simulink model "Q15"  (R2016b)
settings: Solver=VariableStepAuto  StartTime=0.0  StopTime=10.0  RelTol=1e-3
libraries: simulink x1
settings Model: Creator=AKSHAY JP PAWAR  LastModifiedBy=AKSHAY JP PAWAR
settings DataIOCC: ReturnWorkspaceOutputs=on
settings SFSimCC: SimUseLocalCustomCode=on
settings RTWCC: RTWUseLocalCustomCode=on

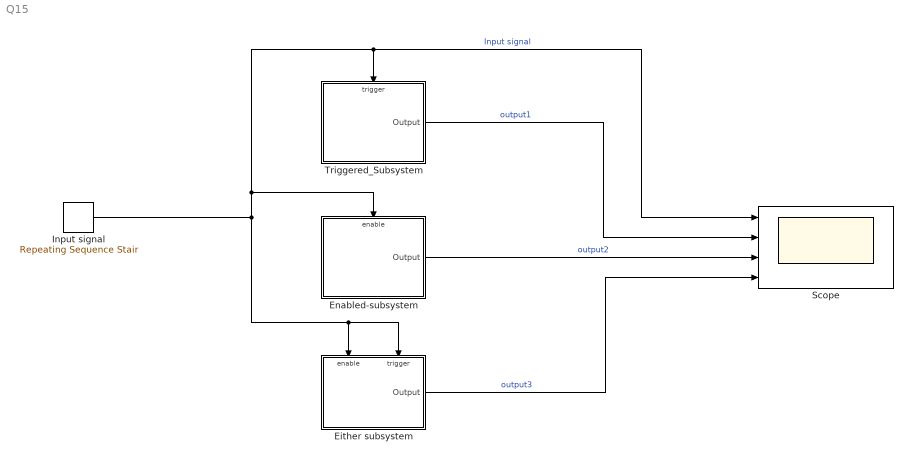
== system Q15 ==
  Either subsystem : Subsystem
  Enabled-subsystem : Subsystem
  Input signal : simulink/Sources/Repeating Sequence Stair  OutValues=[0 1 1 0 0].'  tsamp=-1  OutMin=[]  OutMax=[]  OutDataTypeStr=double  OutputDataTypeScalingMode=double  OutDataType=fixdt(0,8)  ConRadixGroup=Best Precision: Vector-wise  OutScaling=2^-12
  Scope : Scope  NumInputPorts=4
  Triggered_Subsystem : Subsystem
  wires:
  Triggered_Subsystem/1(Output) -> Scope/2  "output1"
  Enabled-subsystem/1(Output) -> Scope/3  "output2"
  Either subsystem/1(Output) -> Scope/4  "output3"
  Input signal/1 -> Enabled-subsystem/Enable, Triggered_Subsystem/Trigger, Scope/1, Either subsystem/Enable, Either subsystem/Trigger  "Input signal"

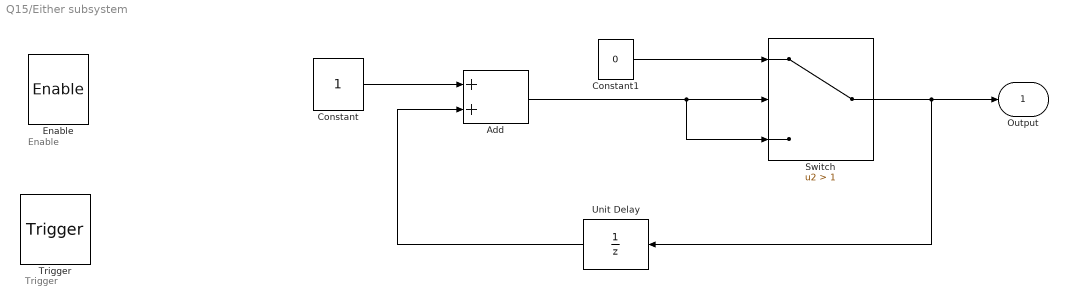
== system Q15/Either subsystem ==
  note: Trigger
  note: Enable
  Enable : EnablePort
  Trigger : TriggerPort  VariantControl=Variant  PortDimensions=1
  Add : Sum
  Constant : Constant
  Constant1 : Constant  Value=0
  Switch : Switch  Criteria=u2 > Threshold  Threshold=1
  Unit Delay : UnitDelay  SampleTime=-1  HasFrameUpgradeWarning=on
  Output : Outport
  wires:
  Add/1 -> Switch/3, Switch/2
  Unit Delay/1 -> Add/2
  Constant/1 -> Add/1
  Constant1/1 -> Switch/1
  Switch/1 -> Unit Delay/1, Output/1

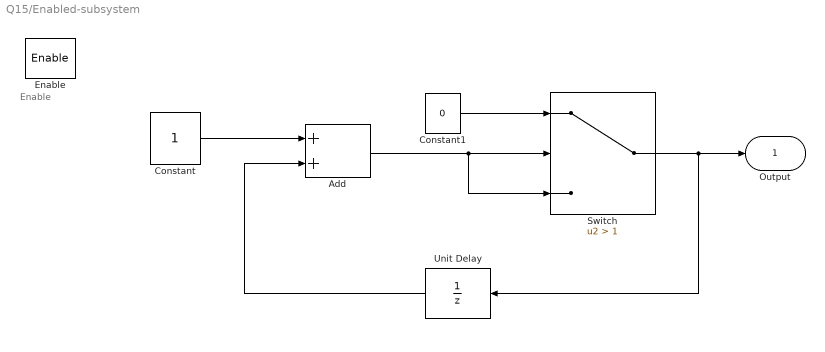
== system Q15/Enabled-subsystem ==
  note: Enable
  Enable : EnablePort
  Add : Sum
  Constant : Constant
  Constant1 : Constant  Value=0
  Switch : Switch  Criteria=u2 > Threshold  Threshold=1
  Unit Delay : UnitDelay  SampleTime=-1  HasFrameUpgradeWarning=on
  Output : Outport
  wires:
  Add/1 -> Switch/3, Switch/2
  Unit Delay/1 -> Add/2
  Constant/1 -> Add/1
  Constant1/1 -> Switch/1
  Switch/1 -> Output/1, Unit Delay/1

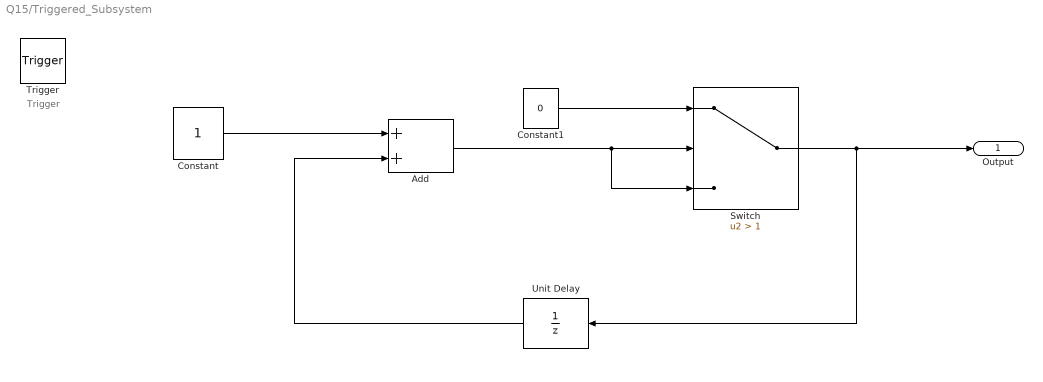
== system Q15/Triggered_Subsystem ==
  note: Trigger
  Trigger : TriggerPort  VariantControl=Variant  PortDimensions=1
  Add : Sum
  Constant : Constant
  Constant1 : Constant  Value=0
  Switch : Switch  Criteria=u2 > Threshold  Threshold=1
  Unit Delay : UnitDelay  SampleTime=-1  HasFrameUpgradeWarning=on
  Output : Outport
  wires:
  Constant1/1 -> Switch/1
  Add/1 -> Switch/3, Switch/2
  Constant/1 -> Add/1
  Switch/1 -> Unit Delay/1, Output/1
  Unit Delay/1 -> Add/2
